simulink model "hwTarget"  (R2020b)
settings: Solver=VariableStepAuto  StartTime=0.0  StopTime=Ts  RelTol=1e-3
InitFcn:
  | evalin('base','pixelcontrolbus');
  | 
  | ROWS = 480;
  | COLS = 752;
  | 
  | OFFSET = 3;
  | imagesToRead = 20;
  | Ts = (imagesToRead + OFFSET) * 2;
  | 
  | inputNums = [1:imagesToRead];
  | 
  | MagThrL = 7;
  | MagThrS = 3;
  | SegMaxLength = 630;
  | 
  | NUM_OF_BITS = 32;
  | MSB = NUM_OF_BITS-1;
  | cap_1 = fixdt(0,NUM_OF_BITS,NUM_OF_BITS-1);
  | cap_2 = fixdt(0,NUM_OF_BITS,NUM_OF_BITS-2);
  | 
  | CORDIC_LUT_DT_1 = fixdt(1, NUM_OF_BITS, NUM_OF_BITS-2);
  | CORDIC_LUT_DT_2 = fixdt(1, NUM_OF_BITS, NUM_OF_BITS-1);
  | CORDIC_LUT_DT_3 = fixdt(1, NUM_OF_BITS, NUM_OF_BITS);
  | CORDIC_LUT_DT_4 = fixdt(1, NUM_OF_BITS, NUM_OF_BITS+1);
  | CORDIC_LUT_DT_5 = fixdt(1, NUM_OF_BITS, NUM_OF_BITS+1);
  | CORDIC_LUT_DT_6 = fixdt(1, NUM_OF_BITS, NUM_OF_BITS+2);
  | CORDIC_LUT_DT_7 = fixdt(1, NUM_OF_BITS, NUM_OF_BITS+3);
  | CORDIC_LUT_DT_8 = fixdt(1, NUM_OF_BITS, NUM_OF_BITS+4);
  | CORDIC_LUT_DT_9 = fixdt(1, NUM_OF_BITS, NUM_OF_BITS+5);
  | CORDIC_LUT_DT_10 = fixdt(1, NUM_OF_BITS, NUM_OF_BITS+6);
  | CORDIC_LUT_DT_11 = fixdt(1, NUM_OF_BITS, NUM_OF_BITS+7);
  | CORDIC_LUT_DT_12 = fixdt(1, NUM_OF_BITS, NUM_OF_BITS+8);
  | 
  | RGB_DT = fixdt(0, 24, 0);
  | GRAY_DT = fixdt(0, 8, 0);
  | THETA_DT = fixdt(1, 16, 13);
  | MAG_DT = fixdt(0, 16, 15);
  | KIRCH_DT = fixdt(0, 12, 0);
undefined symbols (not defined in the file or in its folder): bufferInit, bufferSize
libraries: hdlsllib x86, simulink x6, visionhdlstatistics x4, visionhdlio x2, visionhdlutilities x1
(part 2 of 3)

== system hwTarget/hwTarget/Kirsch Operation North/Kirch Filter North/Kirch Filter ==
  data_in : Inport
  Enable : EnablePort
  Abs : Abs  OutDataTypeStr=fixdt(0,12,0)
  Delay{,1..3,5} (5 alike) : Delay  DelayLength=1
  Gain1 : Gain  Gain=3  OutDataTypeStr=fixdt(0,13,0)
  Multiply : Gain  Gain=5  OutDataTypeStr=fixdt(0,13,0)
  Subtract : Sum  Inputs=+-  OutDataTypeStr=fixdt(1,13,0)
  Sum : Sum  Inputs=+  OutDataTypeStr=fixdt(0,10,0)
  Sum1 : Sum  Inputs=+  OutDataTypeStr=fixdt(0,11,0)
  slicer : Subsystem
  Out1 : Outport
  wires:
  slicer/2(nThrees) -> Sum1/1
  slicer/1(Fives) -> Sum/1
  Sum/1 -> Delay1/1
  Delay/1 -> Gain1/1
  Delay1/1 -> Multiply/1
  Subtract/1 -> Abs/1
  Sum1/1 -> Delay/1
  Abs/1 -> Delay5/1
  Delay2/1 -> Subtract/2
  Gain1/1 -> Delay2/1
  Delay3/1 -> Subtract/1
  Multiply/1 -> Delay3/1
  data_in/1 -> slicer/1(data_in)
  Delay5/1 -> Out1/1

== system hwTarget/hwTarget/Kirsch Operation North/Statistical Analysis/Latch ==
  note: Latch (Active low rst)
      | Ethan Tola
      | 04/03/2021
  D : Inport
  en : Inport  Port=2  OutMin=[0]  OutMax=[1]
  rstn : Inport  Port=3
  Constant : Constant  Value=0  OutDataTypeStr=Inherit: Inherit via back propagation  SampleTime=-1
  Data Type Duplicate : DataTypeDuplicate
  Memory : Memory  InheritSampleTime=on
  Switch : Switch  Criteria=u2 > Threshold
  Switch1 : Switch  Criteria=u2 > Threshold
  Q : Outport
  wires:
  Memory/1 -> Switch/3
  Switch/1 -> Data Type Duplicate/1, Switch1/1, Memory/1
  en/1 -> Switch/2
  D/1 -> Switch/1
  Switch1/1 -> Q/1
  rstn/1 -> Switch1/2
  Constant/1 -> Switch1/3, Data Type Duplicate/2

== system hwTarget/hwTarget/Kirsch Operation North/Statistical Analysis/Latch1 ==
  note: Latch (Active low rst)
      | Ethan Tola
      | 04/03/2021
  D : Inport
  en : Inport  Port=2  OutMin=[0]  OutMax=[1]
  rstn : Inport  Port=3
  Constant : Constant  Value=0  OutDataTypeStr=Inherit: Inherit via back propagation  SampleTime=-1
  Data Type Duplicate : DataTypeDuplicate
  Memory : Memory  InheritSampleTime=on
  Switch : Switch  Criteria=u2 > Threshold
  Switch1 : Switch  Criteria=u2 > Threshold
  Q : Outport
  wires:
  Memory/1 -> Switch/3
  Switch/1 -> Data Type Duplicate/1, Switch1/1, Memory/1
  en/1 -> Switch/2
  D/1 -> Switch/1
  Switch1/1 -> Q/1
  rstn/1 -> Switch1/2
  Constant/1 -> Switch1/3, Data Type Duplicate/2

== system hwTarget/hwTarget/Kirsch Operation Northwest/Binarize/Subsystem ==
  pixel : Inport
  mean : Inport  Port=2
  stddev : Inport  Port=3
  magThrL : Inport  Port=4
  magThrS : Inport  Port=5
  Enable : EnablePort
  Comparator : RelationalOperator  Operator=>  OutDataTypeStr=boolean  RndMeth=Simplest
  Comparator1 : RelationalOperator  Operator=>  OutDataTypeStr=boolean  RndMeth=Simplest
  Delay : Delay  DelayLength=1
  Delay1 : Delay  DelayLength=1
  Delay2 : Delay  DelayLength=1
  MagThrL : Subsystem
  MagThrS : Subsystem
  Out1 : Outport
  Out2 : Outport  Port=2
  wires:
  pixel/1 -> Delay2/1
  MagThrL/1(thresh) -> Delay1/1
  magThrS/1 -> MagThrS/3(dev_step)
  MagThrS/1(thresh) -> Delay/1
  magThrL/1 -> MagThrL/3(dev_step)
  mean/1 -> MagThrS/1(mean), MagThrL/1(mean)
  stddev/1 -> MagThrS/2(stddev), MagThrL/2(stddev)
  Comparator1/1 -> Out2/1
  Comparator/1 -> Out1/1
  Delay/1 -> Comparator1/2
  Delay1/1 -> Comparator/2
  Delay2/1 -> Comparator1/1, Comparator/1

== system hwTarget/hwTarget/Kirsch Operation Northwest/Kirch Filter North-West/Kirch Filter ==
  data_in : Inport
  Enable : EnablePort
  Abs : Abs  OutDataTypeStr=fixdt(0,12,0)
  Delay{,1..3,5} (5 alike) : Delay  DelayLength=1
  Gain1 : Gain  Gain=3  OutDataTypeStr=fixdt(0,13,0)
  Multiply : Gain  Gain=5  OutDataTypeStr=fixdt(0,13,0)
  Subtract : Sum  Inputs=+-  OutDataTypeStr=fixdt(1,13,0)
  Sum : Sum  Inputs=+  OutDataTypeStr=fixdt(0,10,0)
  Sum1 : Sum  Inputs=+  OutDataTypeStr=fixdt(0,11,0)
  slicer : Subsystem
  Out1 : Outport
  wires:
  Sum/1 -> Delay1/1
  Subtract/1 -> Abs/1
  Gain1/1 -> Delay2/1
  Multiply/1 -> Delay3/1
  slicer/2(nThrees) -> Sum1/1
  Sum1/1 -> Delay/1
  Delay3/1 -> Subtract/1
  Delay/1 -> Gain1/1
  Delay1/1 -> Multiply/1
  Abs/1 -> Delay5/1
  slicer/1(Fives) -> Sum/1
  Delay2/1 -> Subtract/2
  data_in/1 -> slicer/1(data_in)
  Delay5/1 -> Out1/1

== system hwTarget/hwTarget/Kirsch Operation Northwest/Statistical Analysis/Latch ==
  note: Latch (Active low rst)
      | Ethan Tola
      | 04/03/2021
  D : Inport
  en : Inport  Port=2  OutMin=[0]  OutMax=[1]
  rstn : Inport  Port=3
  Constant : Constant  Value=0  OutDataTypeStr=Inherit: Inherit via back propagation  SampleTime=-1
  Data Type Duplicate : DataTypeDuplicate
  Memory : Memory  InheritSampleTime=on
  Switch : Switch  Criteria=u2 > Threshold
  Switch1 : Switch  Criteria=u2 > Threshold
  Q : Outport
  wires:
  Memory/1 -> Switch/3
  Switch/1 -> Data Type Duplicate/1, Switch1/1, Memory/1
  en/1 -> Switch/2
  D/1 -> Switch/1
  Switch1/1 -> Q/1
  rstn/1 -> Switch1/2
  Constant/1 -> Switch1/3, Data Type Duplicate/2

== system hwTarget/hwTarget/Kirsch Operation Northwest/Statistical Analysis/Latch1 ==
  note: Latch (Active low rst)
      | Ethan Tola
      | 04/03/2021
  D : Inport
  en : Inport  Port=2  OutMin=[0]  OutMax=[1]
  rstn : Inport  Port=3
  Constant : Constant  Value=0  OutDataTypeStr=Inherit: Inherit via back propagation  SampleTime=-1
  Data Type Duplicate : DataTypeDuplicate
  Memory : Memory  InheritSampleTime=on
  Switch : Switch  Criteria=u2 > Threshold
  Switch1 : Switch  Criteria=u2 > Threshold
  Q : Outport
  wires:
  Memory/1 -> Switch/3
  Switch/1 -> Data Type Duplicate/1, Switch1/1, Memory/1
  en/1 -> Switch/2
  D/1 -> Switch/1
  Switch1/1 -> Q/1
  rstn/1 -> Switch1/2
  Constant/1 -> Switch1/3, Data Type Duplicate/2

== system hwTarget/hwTarget/Kirsch Operation Southwest/Binarize/Subsystem ==
  pixel : Inport
  mean : Inport  Port=2
  stddev : Inport  Port=3
  magThrL : Inport  Port=4
  magThrS : Inport  Port=5
  Enable : EnablePort
  Comparator : RelationalOperator  Operator=>  OutDataTypeStr=boolean  RndMeth=Simplest
  Comparator1 : RelationalOperator  Operator=>  OutDataTypeStr=boolean  RndMeth=Simplest
  Delay : Delay  DelayLength=1
  Delay1 : Delay  DelayLength=1
  Delay2 : Delay  DelayLength=1
  MagThrL : Subsystem
  MagThrS : Subsystem
  Out1 : Outport
  Out2 : Outport  Port=2
  wires:
  pixel/1 -> Delay2/1
  MagThrL/1(thresh) -> Delay1/1
  magThrS/1 -> MagThrS/3(dev_step)
  MagThrS/1(thresh) -> Delay/1
  magThrL/1 -> MagThrL/3(dev_step)
  mean/1 -> MagThrS/1(mean), MagThrL/1(mean)
  stddev/1 -> MagThrS/2(stddev), MagThrL/2(stddev)
  Comparator1/1 -> Out2/1
  Comparator/1 -> Out1/1
  Delay/1 -> Comparator1/2
  Delay1/1 -> Comparator/2
  Delay2/1 -> Comparator1/1, Comparator/1

== system hwTarget/hwTarget/Kirsch Operation Southwest/Kirch Filter South-West/Subsystem ==
  data_in : Inport
  Enable : EnablePort
  Abs : Abs  OutDataTypeStr=fixdt(0,12,0)
  Delay{,1..3,5} (5 alike) : Delay  DelayLength=1
  Gain1 : Gain  Gain=3  OutDataTypeStr=fixdt(0,13,0)
  Multiply : Gain  Gain=5  OutDataTypeStr=fixdt(0,13,0)
  Subtract : Sum  Inputs=+-  OutDataTypeStr=fixdt(1,13,0)
  Sum : Sum  Inputs=+  OutDataTypeStr=fixdt(0,10,0)
  Sum1 : Sum  Inputs=+  OutDataTypeStr=fixdt(0,11,0)
  slicer : Subsystem
  Out1 : Outport
  wires:
  Delay1/1 -> Multiply/1
  slicer/2(nThrees) -> Sum1/1
  Delay/1 -> Gain1/1
  Gain1/1 -> Delay2/1
  Delay3/1 -> Subtract/1
  Subtract/1 -> Abs/1
  slicer/1(Fives) -> Sum/1
  Multiply/1 -> Delay3/1
  Abs/1 -> Delay5/1
  Delay5/1 -> Out1/1
  Delay2/1 -> Subtract/2
  Sum/1 -> Delay1/1
  Sum1/1 -> Delay/1
  data_in/1 -> slicer/1(data_in)

== system hwTarget/hwTarget/Kirsch Operation Southwest/Statistical Analysis/Latch ==
  note: Latch (Active low rst)
      | Ethan Tola
      | 04/03/2021
  D : Inport
  en : Inport  Port=2  OutMin=[0]  OutMax=[1]
  rstn : Inport  Port=3
  Constant : Constant  Value=0  OutDataTypeStr=Inherit: Inherit via back propagation  SampleTime=-1
  Data Type Duplicate : DataTypeDuplicate
  Memory : Memory  InheritSampleTime=on
  Switch : Switch  Criteria=u2 > Threshold
  Switch1 : Switch  Criteria=u2 > Threshold
  Q : Outport
  wires:
  Memory/1 -> Switch/3
  Switch/1 -> Data Type Duplicate/1, Switch1/1, Memory/1
  en/1 -> Switch/2
  D/1 -> Switch/1
  Switch1/1 -> Q/1
  rstn/1 -> Switch1/2
  Constant/1 -> Switch1/3, Data Type Duplicate/2

== system hwTarget/hwTarget/Kirsch Operation Southwest/Statistical Analysis/Latch1 ==
  note: Latch (Active low rst)
      | Ethan Tola
      | 04/03/2021
  D : Inport
  en : Inport  Port=2  OutMin=[0]  OutMax=[1]
  rstn : Inport  Port=3
  Constant : Constant  Value=0  OutDataTypeStr=Inherit: Inherit via back propagation  SampleTime=-1
  Data Type Duplicate : DataTypeDuplicate
  Memory : Memory  InheritSampleTime=on
  Switch : Switch  Criteria=u2 > Threshold
  Switch1 : Switch  Criteria=u2 > Threshold
  Q : Outport
  wires:
  Memory/1 -> Switch/3
  Switch/1 -> Data Type Duplicate/1, Switch1/1, Memory/1
  en/1 -> Switch/2
  D/1 -> Switch/1
  Switch1/1 -> Q/1
  rstn/1 -> Switch1/2
  Constant/1 -> Switch1/3, Data Type Duplicate/2

== system hwTarget/hwTarget/Kirsch Operation West/Binarize/Subsystem ==
  pixel : Inport
  mean : Inport  Port=2
  stddev : Inport  Port=3
  magThrL : Inport  Port=4
  magThrS : Inport  Port=5
  Enable : EnablePort
  Comparator : RelationalOperator  Operator=>  OutDataTypeStr=boolean  RndMeth=Simplest
  Comparator1 : RelationalOperator  Operator=>  OutDataTypeStr=boolean  RndMeth=Simplest
  Delay : Delay  DelayLength=1
  Delay1 : Delay  DelayLength=1
  Delay2 : Delay  DelayLength=1
  MagThrL : Subsystem
  MagThrS : Subsystem
  Out1 : Outport
  Out2 : Outport  Port=2
  wires:
  pixel/1 -> Delay2/1
  MagThrL/1(thresh) -> Delay1/1
  magThrS/1 -> MagThrS/3(dev_step)
  MagThrS/1(thresh) -> Delay/1
  magThrL/1 -> MagThrL/3(dev_step)
  mean/1 -> MagThrS/1(mean), MagThrL/1(mean)
  stddev/1 -> MagThrS/2(stddev), MagThrL/2(stddev)
  Comparator1/1 -> Out2/1
  Comparator/1 -> Out1/1
  Delay/1 -> Comparator1/2
  Delay1/1 -> Comparator/2
  Delay2/1 -> Comparator1/1, Comparator/1

== system hwTarget/hwTarget/Kirsch Operation West/Kirch Filter West/Subsystem ==
  data_in : Inport
  Enable : EnablePort
  Abs : Abs  OutDataTypeStr=fixdt(0,12,0)
  Delay{,1..3,5} (5 alike) : Delay  DelayLength=1
  Gain1 : Gain  Gain=3  OutDataTypeStr=fixdt(0,13,0)
  Multiply : Gain  Gain=5  OutDataTypeStr=fixdt(0,13,0)
  Subtract : Sum  Inputs=+-  OutDataTypeStr=fixdt(1,13,0)
  Sum : Sum  Inputs=+  OutDataTypeStr=fixdt(0,10,0)
  Sum1 : Sum  Inputs=+  OutDataTypeStr=fixdt(0,11,0)
  slicer : Subsystem
  Out1 : Outport
  wires:
  Subtract/1 -> Abs/1
  Abs/1 -> Delay5/1
  Delay2/1 -> Subtract/2
  Multiply/1 -> Delay3/1
  Delay3/1 -> Subtract/1
  Delay1/1 -> Multiply/1
  slicer/1(Fives) -> Sum/1
  Delay/1 -> Gain1/1
  Sum1/1 -> Delay/1
  slicer/2(nThrees) -> Sum1/1
  Sum/1 -> Delay1/1
  Delay5/1 -> Out1/1
  Gain1/1 -> Delay2/1
  data_in/1 -> slicer/1(data_in)

== system hwTarget/hwTarget/Kirsch Operation West/Statistical Analysis/Latch ==
  note: Latch (Active low rst)
      | Ethan Tola
      | 04/03/2021
  D : Inport
  en : Inport  Port=2  OutMin=[0]  OutMax=[1]
  rstn : Inport  Port=3
  Constant : Constant  Value=0  OutDataTypeStr=Inherit: Inherit via back propagation  SampleTime=-1
  Data Type Duplicate : DataTypeDuplicate
  Memory : Memory  InheritSampleTime=on
  Switch : Switch  Criteria=u2 > Threshold
  Switch1 : Switch  Criteria=u2 > Threshold
  Q : Outport
  wires:
  Memory/1 -> Switch/3
  Switch/1 -> Data Type Duplicate/1, Switch1/1, Memory/1
  en/1 -> Switch/2
  D/1 -> Switch/1
  Switch1/1 -> Q/1
  rstn/1 -> Switch1/2
  Constant/1 -> Switch1/3, Data Type Duplicate/2

== system hwTarget/hwTarget/Kirsch Operation West/Statistical Analysis/Latch1 ==
  note: Latch (Active low rst)
      | Ethan Tola
      | 04/03/2021
  D : Inport
  en : Inport  Port=2  OutMin=[0]  OutMax=[1]
  rstn : Inport  Port=3
  Constant : Constant  Value=0  OutDataTypeStr=Inherit: Inherit via back propagation  SampleTime=-1
  Data Type Duplicate : DataTypeDuplicate
  Memory : Memory  InheritSampleTime=on
  Switch : Switch  Criteria=u2 > Threshold
  Switch1 : Switch  Criteria=u2 > Threshold
  Q : Outport
  wires:
  Memory/1 -> Switch/3
  Switch/1 -> Data Type Duplicate/1, Switch1/1, Memory/1
  en/1 -> Switch/2
  D/1 -> Switch/1
  Switch1/1 -> Q/1
  rstn/1 -> Switch1/2
  Constant/1 -> Switch1/3, Data Type Duplicate/2

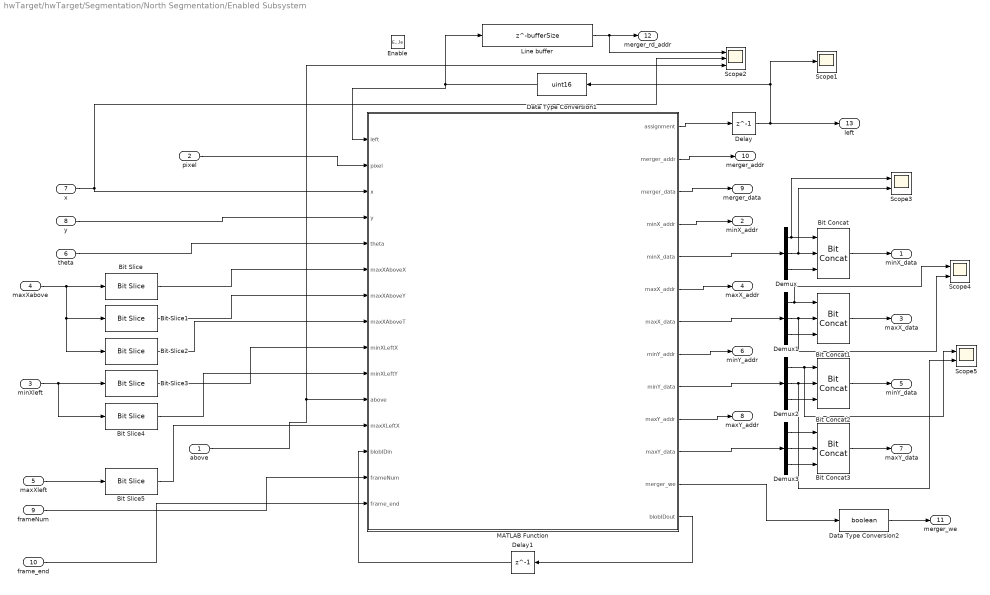
== system hwTarget/hwTarget/Segmentation/North Segmentation/Enabled Subsystem ==
  above : Inport
  pixel : Inport  Port=2
  minXleft : Inport  Port=3
  maxXabove : Inport  Port=4
  maxXleft : Inport  Port=5
  theta : Inport  Port=6
  x : Inport  Port=7
  y : Inport  Port=8
  frameNum : Inport  Port=9
  frame_end : Inport  Port=10
  Enable : EnablePort
  Bit Concat{,1..3} (4 alike) : hdlsllib/Logic and Bit Operations/Bit Concat  numInputs=3
  Bit Slice : hdlsllib/Logic and Bit Operations/Bit Slice  lidx=47  ridx=32
      settings: SourceProductBaseCode=SL
  Bit Slice1 : hdlsllib/Logic and Bit Operations/Bit Slice  lidx=31  ridx=16
      settings: SourceProductBaseCode=SL
  Bit Slice2 : hdlsllib/Logic and Bit Operations/Bit Slice  lidx=15  ridx=0
      settings: SourceProductBaseCode=SL
  Bit Slice3 : hdlsllib/Logic and Bit Operations/Bit Slice  lidx=47  ridx=32
      settings: SourceProductBaseCode=SL
  Bit Slice4 : hdlsllib/Logic and Bit Operations/Bit Slice  lidx=31  ridx=16
      settings: SourceProductBaseCode=SL
  Bit Slice5 : hdlsllib/Logic and Bit Operations/Bit Slice  lidx=47  ridx=32
      settings: SourceProductBaseCode=SL
  Data Type Conversion1 : DataTypeConversion  OutDataTypeStr=uint16
  Data Type Conversion2 : DataTypeConversion  OutDataTypeStr=boolean
  Delay : Delay  DelayLength=1  InitialCondition=0
  Delay1 : Delay  DelayLength=1  InitialCondition=1
  Demux{,1..3} (4 alike) : Demux  Outputs=3
  Line buffer : Delay  DelayLength=bufferSize  InitialCondition=bufferInit
  MATLAB Function : MATLAB Function  TreatAsAtomicUnit=on
  Scope1 : Scope
  Scope2 : Scope  NumInputPorts=3
  Scope3 : Scope  NumInputPorts=2
  Scope4 : Scope  NumInputPorts=2
  Scope5 : Scope  NumInputPorts=2
  minX_data : Outport  InitialOutput=0
  minX_addr : Outport  Port=2  InitialOutput=0
  maxX_data : Outport  Port=3  InitialOutput=0
  maxX_addr : Outport  Port=4  InitialOutput=0
  minY_data : Outport  Port=5  InitialOutput=0
  minY_addr : Outport  Port=6  InitialOutput=0
  maxY_data : Outport  Port=7  InitialOutput=0
  maxY_addr : Outport  Port=8  InitialOutput=0
  merger_data : Outport  Port=9  InitialOutput=0
  merger_addr : Outport  Port=10  InitialOutput=0
  merger_we : Outport  Port=11  InitialOutput=0
  merger_rd_addr : Outport  Port=12  InitialOutput=0
  left : Outport  Port=13  InitialOutput=0
  wires:
  Line buffer/1 -> Scope2/1, merger_rd_addr/1
  MATLAB Function/6(maxX_addr) -> maxX_addr/1
  MATLAB Function/4(minX_addr) -> minX_addr/1
  MATLAB Function/8(minY_addr) -> minY_addr/1
  MATLAB Function/10(maxY_addr) -> maxY_addr/1
  MATLAB Function/2(merger_addr) -> merger_addr/1
  Delay/1 -> Scope1/1, Data Type Conversion1/1, left/1
  MATLAB Function/1(assignment) -> Delay/1
  MATLAB Function/12(merger_we) -> Data Type Conversion2/1
  maxXabove/1 -> Bit Slice2/1, Bit Slice1/1, Bit Slice/1
  MATLAB Function/5(minX_data) -> Demux/1
  Bit Concat/1 -> minX_data/1
  Demux/1 -> Scope3/1, Bit Concat/1
  Demux/2 -> Scope3/2, Bit Concat/2
  Demux/3 -> Bit Concat/3
  MATLAB Function/7(maxX_data) -> Demux1/1
  Demux1/3 -> Bit Concat1/3
  Demux1/1 -> Scope4/1, Bit Concat1/1
  Demux1/2 -> Scope4/2, Bit Concat1/2
  Bit Concat1/1 -> maxX_data/1
  MATLAB Function/9(minY_data) -> Demux2/1
  Demux2/3 -> Bit Concat2/3
  Demux2/1 -> Scope5/1, Bit Concat2/1
  Demux2/2 -> Scope5/2, Bit Concat2/2
  Bit Concat2/1 -> minY_data/1
  MATLAB Function/11(maxY_data) -> Demux3/1
  Demux3/3 -> Bit Concat3/3
  Demux3/1 -> Bit Concat3/1
  Demux3/2 -> Bit Concat3/2
  Bit Concat3/1 -> maxY_data/1
  Data Type Conversion1/1 -> MATLAB Function/1(left), Line buffer/1
  pixel/1 -> MATLAB Function/2(pixel)
  x/1 -> Scope2/2, MATLAB Function/3(x)
  y/1 -> MATLAB Function/4(y)
  theta/1 -> MATLAB Function/5(theta)
  Bit Slice/1 -> MATLAB Function/6(maxXAboveX)
  Bit Slice1/1 -> MATLAB Function/7(maxXAboveY)
  Bit Slice2/1 -> MATLAB Function/8(maxXAboveT)
  Bit Slice3/1 -> MATLAB Function/9(minXLeftX)
  Bit Slice4/1 -> MATLAB Function/10(minXLeftY)
  Bit Slice5/1 -> MATLAB Function/12(maxXLeftX)
  above/1 -> Scope2/3, MATLAB Function/11(above)
  Data Type Conversion2/1 -> merger_we/1
  MATLAB Function/3(merger_data) -> merger_data/1
  Delay1/1 -> MATLAB Function/13(blobIDin)
  MATLAB Function/13(blobIDout) -> Delay1/1
  frameNum/1 -> MATLAB Function/14(frameNum)
  maxXleft/1 -> Bit Slice5/1
  minXleft/1 -> Bit Slice4/1, Bit Slice3/1
  frame_end/1 -> MATLAB Function/15(frame_end)

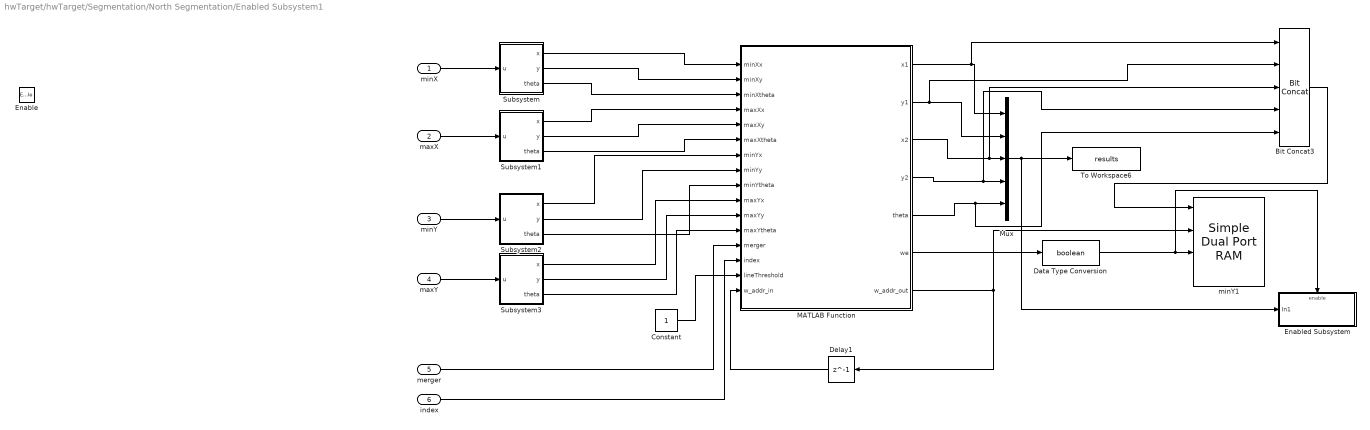
== system hwTarget/hwTarget/Segmentation/North Segmentation/Enabled Subsystem1 ==
  minX : Inport
  maxX : Inport  Port=2
  minY : Inport  Port=3
  maxY : Inport  Port=4
  merger : Inport  Port=5
  index : Inport  Port=6
  Enable : EnablePort
  Bit Concat3 : hdlsllib/Logic and Bit Operations/Bit Concat  numInputs=5
  Constant : Constant  OutDataTypeStr=uint16  SampleTime=-1
  Data Type Conversion : DataTypeConversion  OutDataTypeStr=boolean
  Delay1 : Delay  DelayLength=1  InitialCondition=0
  Enabled Subsystem : Subsystem  TreatAsAtomicUnit=on
  MATLAB Function : MATLAB Function  TreatAsAtomicUnit=on
  Mux : Mux  Inputs=5
  Subsystem : Subsystem
  Subsystem1 : Subsystem
  Subsystem2 : Subsystem
  Subsystem3 : Subsystem
  To Workspace6 : ToWorkspace  VariableName=results  SaveFormat=Timeseries  SampleTime=-1
  minY1 : hdlsllib/HDL RAMs/Simple Dual Port RAM  ram_size=16
      settings: SourceProductBaseCode=SL
  wires:
  minX/1 -> Subsystem/1(u)
  Subsystem/1(x) -> MATLAB Function/1(minXx)
  Subsystem/2(y) -> MATLAB Function/2(minXy)
  maxX/1 -> Subsystem1/1(u)
  minY/1 -> Subsystem2/1(u)
  Subsystem/3(theta) -> MATLAB Function/3(minXtheta)
  Subsystem1/1(x) -> MATLAB Function/4(maxXx)
  Subsystem1/2(y) -> MATLAB Function/5(maxXy)
  Subsystem1/3(theta) -> MATLAB Function/6(maxXtheta)
  Subsystem2/1(x) -> MATLAB Function/7(minYx)
  Subsystem2/2(y) -> MATLAB Function/8(minYy)
  Subsystem2/3(theta) -> MATLAB Function/9(minYtheta)
  maxY/1 -> Subsystem3/1(u)
  Subsystem3/1(x) -> MATLAB Function/10(maxYx)
  Subsystem3/2(y) -> MATLAB Function/11(maxYy)
  Subsystem3/3(theta) -> MATLAB Function/12(maxYtheta)
  merger/1 -> MATLAB Function/13(merger)
  index/1 -> MATLAB Function/14(index)
  Constant/1 -> MATLAB Function/15(lineThreshold)
  MATLAB Function/1(x1) -> Bit Concat3/1, Mux/1
  MATLAB Function/2(y1) -> Bit Concat3/2, Mux/2
  MATLAB Function/3(x2) -> Bit Concat3/3, Mux/3
  MATLAB Function/4(y2) -> Bit Concat3/4, Mux/4
  MATLAB Function/5(theta) -> Bit Concat3/5, Mux/5
  Mux/1 -> Enabled Subsystem/1(In1), To Workspace6/1
  MATLAB Function/7(w_addr_out) -> minY1/2, Delay1/1
  Delay1/1 -> MATLAB Function/16(w_addr_in)
  MATLAB Function/6(we) -> Data Type Conversion/1
  Bit Concat3/1 -> minY1/1
  Data Type Conversion/1 -> Enabled Subsystem/Enable, minY1/3

== system hwTarget/hwTarget/Segmentation/North Segmentation/Subsystem1 ==
  enable : Inport
  Constant : Constant  OutDataTypeStr=fixdt(0,10,0)  SampleTime=-1
  Delay2 : Delay  DelayLength=1  InitialCondition=1  ShowEnablePort=on
      settings: InputPortMap=u0,e6
  Sum : Sum  Inputs=|++  OutDataTypeStr=uint16
  counter : Outport
  wires:
  enable/1 -> Delay2/2
  Delay2/1 -> Sum/1
  Constant/1 -> Sum/2
  Sum/1 -> Delay2/1, counter/1  "blobID"

== system hwTarget/hwTarget/Segmentation/North Segmentation/Subsystem2 ==
  reset : Inport
  Constant : Constant  OutDataTypeStr=fixdt(0,10,0)  SampleTime=-1
  Delay2 : Delay  DelayLength=1  InitialCondition=0  ExternalReset=Level
      settings: InputPortMap=u0,r5
  Sum : Sum  Inputs=|++  OutDataTypeStr=uint16
  counter : Outport
  wires:
  reset/1 -> Delay2/2
  Delay2/1 -> Sum/1
  Constant/1 -> Sum/2
  Sum/1 -> Delay2/1, counter/1  "blobID"

== system hwTarget/hwTarget/Segmentation/North Segmentation/Subsystem3 ==
  reset : Inport
  Constant : Constant  OutDataTypeStr=fixdt(0,10,0)  SampleTime=-1
  Delay2 : Delay  DelayLength=1  InitialCondition=0  ExternalReset=Level
      settings: InputPortMap=u0,r5
  Sum : Sum  Inputs=|++  OutDataTypeStr=uint16
  counter : Outport
  wires:
  Sum/1 -> counter/1, Delay2/1  "blobID"
  Constant/1 -> Sum/2
  Delay2/1 -> Sum/1
  reset/1 -> Delay2/2

== system hwTarget/hwTarget/Segmentation/North Segmentation/maxXWriteSwitch ==
  valid : Inport
  data_in : Inport  Port=2
  addr_in : Inport  Port=3
  we_in : Inport  Port=4
  Constant2 : Constant  OutDataTypeStr=boolean  SampleTime=-1
  Constant3 : Constant  Value=0  OutDataTypeStr=boolean  SampleTime=-1
  Counter Limited : simulink/Sources/Counter Limited  uplimit=1023  tsamp=-1
  Index Vector : MultiPortSwitch  DataPortOrder=Zero-based contiguous  Inputs=2  zeroidx=on
  Index Vector1 : MultiPortSwitch  DataPortOrder=Zero-based contiguous  Inputs=2  zeroidx=on
  Index Vector2 : MultiPortSwitch  DataPortOrder=Zero-based contiguous  Inputs=2  zeroidx=on
  data_out : Outport
  addr_out : Outport  Port=2
  we : Outport  Port=3
  wires:
  Constant2/1 -> Index Vector2/2
  Counter Limited/1 -> Index Vector1/2
  Constant3/1 -> Index Vector/2
  valid/1 -> Index Vector/1, Index Vector1/1, Index Vector2/1
  we_in/1 -> Index Vector2/3
  Index Vector2/1 -> we/1
  data_in/1 -> Index Vector/3
  addr_in/1 -> Index Vector1/3
  Index Vector1/1 -> addr_out/1
  Index Vector/1 -> data_out/1

== system hwTarget/hwTarget/Segmentation/North Segmentation/maxYWriteSwitch ==
  valid : Inport
  data_in : Inport  Port=2
  addr_in : Inport  Port=3
  we_in : Inport  Port=4
  Constant2 : Constant  OutDataTypeStr=boolean  SampleTime=-1
  Constant3 : Constant  Value=0  OutDataTypeStr=boolean  SampleTime=-1
  Counter Limited : simulink/Sources/Counter Limited  uplimit=1023  tsamp=-1
  Index Vector : MultiPortSwitch  DataPortOrder=Zero-based contiguous  Inputs=2  zeroidx=on
  Index Vector1 : MultiPortSwitch  DataPortOrder=Zero-based contiguous  Inputs=2  zeroidx=on
  Index Vector2 : MultiPortSwitch  DataPortOrder=Zero-based contiguous  Inputs=2  zeroidx=on
  data_out : Outport
  addr_out : Outport  Port=2
  we : Outport  Port=3
  wires:
  Constant2/1 -> Index Vector2/2
  Counter Limited/1 -> Index Vector1/2
  Constant3/1 -> Index Vector/2
  valid/1 -> Index Vector/1, Index Vector1/1, Index Vector2/1
  we_in/1 -> Index Vector2/3
  Index Vector2/1 -> we/1
  data_in/1 -> Index Vector/3
  addr_in/1 -> Index Vector1/3
  Index Vector1/1 -> addr_out/1
  Index Vector/1 -> data_out/1

== system hwTarget/hwTarget/Segmentation/North Segmentation/minXReadSwitch ==
  valid : Inport
  addr_in1 : Inport  Port=2
  frame_end : Inport  Port=3
  Index Vector : MultiPortSwitch  DataPortOrder=Zero-based contiguous  Inputs=2  zeroidx=on
  Subsystem1 : Subsystem
  addr_out : Outport
  wires:
  valid/1 -> Index Vector/1
  Index Vector/1 -> addr_out/1
  addr_in1/1 -> Index Vector/3
  frame_end/1 -> Subsystem1/1(reset)
  Subsystem1/1(counter) -> Index Vector/2

== system hwTarget/hwTarget/Segmentation/North Segmentation/minXReadSwitch1 ==
  valid : Inport
  addr_in1 : Inport  Port=2
  frame_end : Inport  Port=3
  Index Vector : MultiPortSwitch  DataPortOrder=Zero-based contiguous  Inputs=2  zeroidx=on
  Subsystem1 : Subsystem
  addr_out : Outport
  wires:
  valid/1 -> Index Vector/1
  Index Vector/1 -> addr_out/1
  addr_in1/1 -> Index Vector/3
  frame_end/1 -> Subsystem1/1(reset)
  Subsystem1/1(counter) -> Index Vector/2

== system hwTarget/hwTarget/Segmentation/North Segmentation/minXReadSwitch3 ==
  valid : Inport
  addr_in1 : Inport  Port=2
  frame_end : Inport  Port=3
  Index Vector : MultiPortSwitch  DataPortOrder=Zero-based contiguous  Inputs=2  zeroidx=on
  Subsystem1 : Subsystem
  addr_out : Outport
  wires:
  valid/1 -> Index Vector/1
  Index Vector/1 -> addr_out/1
  addr_in1/1 -> Index Vector/3
  frame_end/1 -> Subsystem1/1(reset)
  Subsystem1/1(counter) -> Index Vector/2

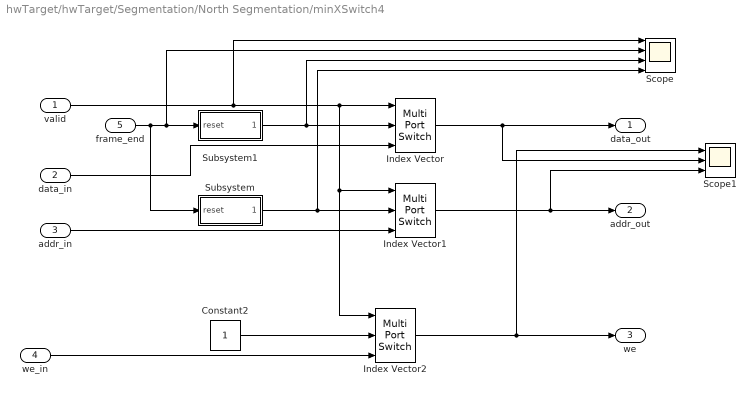
== system hwTarget/hwTarget/Segmentation/North Segmentation/minXSwitch4 ==
  valid : Inport
  data_in : Inport  Port=2
  addr_in : Inport  Port=3
  we_in : Inport  Port=4
  frame_end : Inport  Port=5
  Constant2 : Constant  OutDataTypeStr=boolean  SampleTime=-1
  Index Vector : MultiPortSwitch  DataPortOrder=Zero-based contiguous  Inputs=2  zeroidx=on
  Index Vector1 : MultiPortSwitch  DataPortOrder=Zero-based contiguous  Inputs=2  zeroidx=on
  Index Vector2 : MultiPortSwitch  DataPortOrder=Zero-based contiguous  Inputs=2  zeroidx=on
  Scope : Scope  NumInputPorts=4
  Scope1 : Scope  NumInputPorts=3
  Subsystem : Subsystem
  Subsystem1 : Subsystem
  data_out : Outport
  addr_out : Outport  Port=2
  we : Outport  Port=3
  wires:
  Index Vector/1 -> Scope1/2, data_out/1
  Index Vector1/1 -> Scope1/3, addr_out/1
  addr_in/1 -> Index Vector1/3
  data_in/1 -> Index Vector/3
  Index Vector2/1 -> Scope1/1, we/1
  we_in/1 -> Index Vector2/3
  valid/1 -> Scope/1, Index Vector2/1, Index Vector1/1, Index Vector/1
  Subsystem1/1(counter) -> Scope/3, Index Vector/2
  Subsystem/1(counter) -> Scope/4, Index Vector1/2
  Constant2/1 -> Index Vector2/2
  frame_end/1 -> Subsystem/1(reset), Scope/2, Subsystem1/1(reset)

== system hwTarget/hwTarget/Segmentation/North Segmentation/minXWriteSwitch ==
  valid : Inport
  data_in : Inport  Port=2
  addr_in : Inport  Port=3
  we_in : Inport  Port=4
  Constant2 : Constant  OutDataTypeStr=boolean  SampleTime=-1
  Constant3 : Constant  Value=0  OutDataTypeStr=boolean  SampleTime=-1
  Counter Limited : simulink/Sources/Counter Limited  uplimit=1023  tsamp=-1
  Index Vector : MultiPortSwitch  DataPortOrder=Zero-based contiguous  Inputs=2  zeroidx=on
  Index Vector1 : MultiPortSwitch  DataPortOrder=Zero-based contiguous  Inputs=2  zeroidx=on
  Index Vector2 : MultiPortSwitch  DataPortOrder=Zero-based contiguous  Inputs=2  zeroidx=on
  data_out : Outport
  addr_out : Outport  Port=2
  we : Outport  Port=3
  wires:
  Constant2/1 -> Index Vector2/2
  Counter Limited/1 -> Index Vector1/2
  Constant3/1 -> Index Vector/2
  valid/1 -> Index Vector/1, Index Vector1/1, Index Vector2/1
  we_in/1 -> Index Vector2/3
  Index Vector2/1 -> we/1
  data_in/1 -> Index Vector/3
  addr_in/1 -> Index Vector1/3
  Index Vector1/1 -> addr_out/1
  Index Vector/1 -> data_out/1

== system hwTarget/hwTarget/Segmentation/North Segmentation/minYWriteSwitch ==
  valid : Inport
  data_in : Inport  Port=2
  addr_in : Inport  Port=3
  we_in : Inport  Port=4
  Constant2 : Constant  OutDataTypeStr=boolean  SampleTime=-1
  Constant3 : Constant  Value=0  OutDataTypeStr=boolean  SampleTime=-1
  Counter Limited : simulink/Sources/Counter Limited  uplimit=1023  tsamp=-1
  Index Vector : MultiPortSwitch  DataPortOrder=Zero-based contiguous  Inputs=2  zeroidx=on
  Index Vector1 : MultiPortSwitch  DataPortOrder=Zero-based contiguous  Inputs=2  zeroidx=on
  Index Vector2 : MultiPortSwitch  DataPortOrder=Zero-based contiguous  Inputs=2  zeroidx=on
  data_out : Outport
  addr_out : Outport  Port=2
  we : Outport  Port=3
  wires:
  Index Vector/1 -> data_out/1
  Index Vector1/1 -> addr_out/1
  addr_in/1 -> Index Vector1/3
  data_in/1 -> Index Vector/3
  Index Vector2/1 -> we/1
  we_in/1 -> Index Vector2/3
  valid/1 -> Index Vector2/1, Index Vector1/1, Index Vector/1
  Constant3/1 -> Index Vector/2
  Counter Limited/1 -> Index Vector1/2
  Constant2/1 -> Index Vector2/2

== system hwTarget/hwTarget/CordicAtan/CORDIC Algorithm/Iteration_1/n_zsign ==
  signof : Inport
  base : Inport  Port=2
  Bit Slice : hdlsllib/Logic and Bit Operations/Bit Slice  lidx=MSB  ridx=MSB
      settings: SourceProductBaseCode=SL
  Switch : Switch  Criteria=u2 > Threshold
  Unary Minus : UnaryMinus
  out : Outport
  wires:
  Bit Slice/1 -> Switch/2
  signof/1 -> Bit Slice/1
  base/1 -> Switch/1, Unary Minus/1
  Switch/1 -> out/1
  Unary Minus/1 -> Switch/3

== system hwTarget/hwTarget/CordicAtan/CORDIC Algorithm/Iteration_1/n_zsign1 ==
  signof : Inport
  base : Inport  Port=2
  Bit Slice : hdlsllib/Logic and Bit Operations/Bit Slice  lidx=MSB  ridx=MSB
      settings: SourceProductBaseCode=SL
  Switch : Switch  Criteria=u2 > Threshold
  Unary Minus : UnaryMinus
  out : Outport
  wires:
  Bit Slice/1 -> Switch/2
  signof/1 -> Bit Slice/1
  base/1 -> Switch/1, Unary Minus/1
  Switch/1 -> out/1
  Unary Minus/1 -> Switch/3

== system hwTarget/hwTarget/CordicAtan/CORDIC Algorithm/Iteration_1/zsign ==
  signof : Inport
  base : Inport  Port=2
  Bit Slice : hdlsllib/Logic and Bit Operations/Bit Slice  lidx=MSB  ridx=MSB
      settings: SourceProductBaseCode=SL
  Switch : Switch  Criteria=u2 > Threshold
  Unary Minus : UnaryMinus
  out : Outport
  wires:
  signof/1 -> Bit Slice/1
  Bit Slice/1 -> Switch/2
  base/1 -> Switch/3, Unary Minus/1
  Switch/1 -> out/1
  Unary Minus/1 -> Switch/1

== system hwTarget/hwTarget/CordicAtan/CORDIC Algorithm/Iteration_10/X_Logic ==
  xo : Inport
  yo : Inport  Port=2
  Add2 : Sum
  Bit Shift : hdlsllib/Logic and Bit Operations/Bit Shift  mode=Shift Right Arithmetic  N=9
  zsign : Subsystem
  x : Outport
  wires:
  yo/1 -> zsign/1(signof), Bit Shift/1
  Bit Shift/1 -> zsign/2(base)
  xo/1 -> Add2/1
  Add2/1 -> x/1
  zsign/1(out) -> Add2/2  "xo"

== system hwTarget/hwTarget/CordicAtan/CORDIC Algorithm/Iteration_10/Y_Logic ==
  xo : Inport
  yo : Inport  Port=2
  Add1 : Sum
  Bit Shift : hdlsllib/Logic and Bit Operations/Bit Shift  mode=Shift Right Arithmetic  N=9
  n_zsign : Subsystem
  y : Outport
  wires:
  Bit Shift/1 -> n_zsign/2(base)
  n_zsign/1(out) -> Add1/2
  Add1/1 -> y/1
  xo/1 -> Bit Shift/1
  yo/1 -> n_zsign/1(signof), Add1/1

== system hwTarget/hwTarget/CordicAtan/CORDIC Algorithm/Iteration_10/n_zsign ==
  signof : Inport
  base : Inport  Port=2
  Bit Slice : hdlsllib/Logic and Bit Operations/Bit Slice  lidx=MSB  ridx=MSB
      settings: SourceProductBaseCode=SL
  Switch : Switch  Criteria=u2 > Threshold
  Unary Minus : UnaryMinus
  out : Outport
  wires:
  Bit Slice/1 -> Switch/2
  signof/1 -> Bit Slice/1
  base/1 -> Switch/1, Unary Minus/1
  Switch/1 -> out/1
  Unary Minus/1 -> Switch/3

== system hwTarget/hwTarget/CordicAtan/CORDIC Algorithm/Iteration_2/X_Logic ==
  xo : Inport
  yo : Inport  Port=2
  Add2 : Sum
  Bit Shift : hdlsllib/Logic and Bit Operations/Bit Shift  mode=Shift Right Arithmetic  N=1
  zsign1 : Subsystem
  x : Outport
  wires:
  yo/1 -> zsign1/1(signof), Bit Shift/1
  Bit Shift/1 -> zsign1/2(base)
  xo/1 -> Add2/1
  Add2/1 -> x/1
  zsign1/1(out) -> Add2/2  "xo"

== system hwTarget/hwTarget/CordicAtan/CORDIC Algorithm/Iteration_2/Y_Logic ==
  xo : Inport
  yo : Inport  Port=2
  Add1 : Sum
  Bit Shift : hdlsllib/Logic and Bit Operations/Bit Shift  mode=Shift Right Arithmetic  N=1
  n_zsign : Subsystem
  y : Outport
  wires:
  Bit Shift/1 -> n_zsign/2(base)
  n_zsign/1(out) -> Add1/2
  Add1/1 -> y/1
  xo/1 -> Bit Shift/1
  yo/1 -> n_zsign/1(signof), Add1/1

== system hwTarget/hwTarget/CordicAtan/CORDIC Algorithm/Iteration_2/n_zsign ==
  signof : Inport
  base : Inport  Port=2
  Bit Slice : hdlsllib/Logic and Bit Operations/Bit Slice  lidx=MSB  ridx=MSB
      settings: SourceProductBaseCode=SL
  Switch : Switch  Criteria=u2 > Threshold
  Unary Minus : UnaryMinus
  out : Outport
  wires:
  Bit Slice/1 -> Switch/2
  signof/1 -> Bit Slice/1
  base/1 -> Switch/1, Unary Minus/1
  Switch/1 -> out/1
  Unary Minus/1 -> Switch/3

== system hwTarget/hwTarget/CordicAtan/CORDIC Algorithm/Iteration_3/X_Logic ==
  xo : Inport
  yo : Inport  Port=2
  Add2 : Sum
  Bit Shift : hdlsllib/Logic and Bit Operations/Bit Shift  mode=Shift Right Arithmetic  N=2
  zsign : Subsystem
  x : Outport
  wires:
  yo/1 -> zsign/1(signof), Bit Shift/1
  Bit Shift/1 -> zsign/2(base)
  xo/1 -> Add2/1
  Add2/1 -> x/1
  zsign/1(out) -> Add2/2  "xo"

== system hwTarget/hwTarget/CordicAtan/CORDIC Algorithm/Iteration_3/Y_Logic ==
  xo : Inport
  yo : Inport  Port=2
  Add1 : Sum
  Bit Shift : hdlsllib/Logic and Bit Operations/Bit Shift  mode=Shift Right Arithmetic  N=2
  n_zsign : Subsystem
  y : Outport
  wires:
  Bit Shift/1 -> n_zsign/2(base)
  n_zsign/1(out) -> Add1/2
  Add1/1 -> y/1
  xo/1 -> Bit Shift/1
  yo/1 -> n_zsign/1(signof), Add1/1

== system hwTarget/hwTarget/CordicAtan/CORDIC Algorithm/Iteration_3/n_zsign ==
  signof : Inport
  base : Inport  Port=2
  Bit Slice : hdlsllib/Logic and Bit Operations/Bit Slice  lidx=MSB  ridx=MSB
      settings: SourceProductBaseCode=SL
  Switch : Switch  Criteria=u2 > Threshold
  Unary Minus : UnaryMinus
  out : Outport
  wires:
  Bit Slice/1 -> Switch/2
  signof/1 -> Bit Slice/1
  base/1 -> Switch/1, Unary Minus/1
  Switch/1 -> out/1
  Unary Minus/1 -> Switch/3

== system hwTarget/hwTarget/CordicAtan/CORDIC Algorithm/Iteration_4/X_Logic ==
  xo : Inport
  yo : Inport  Port=2
  Add2 : Sum
  Bit Shift : hdlsllib/Logic and Bit Operations/Bit Shift  mode=Shift Right Arithmetic  N=3
  zsign : Subsystem
  x : Outport
  wires:
  yo/1 -> zsign/1(signof), Bit Shift/1
  Bit Shift/1 -> zsign/2(base)
  xo/1 -> Add2/1
  Add2/1 -> x/1
  zsign/1(out) -> Add2/2  "xo"

== system hwTarget/hwTarget/CordicAtan/CORDIC Algorithm/Iteration_4/Y_Logic ==
  xo : Inport
  yo : Inport  Port=2
  Add1 : Sum
  Bit Shift : hdlsllib/Logic and Bit Operations/Bit Shift  mode=Shift Right Arithmetic  N=3
  n_zsign : Subsystem
  y : Outport
  wires:
  Bit Shift/1 -> n_zsign/2(base)
  n_zsign/1(out) -> Add1/2
  Add1/1 -> y/1
  xo/1 -> Bit Shift/1
  yo/1 -> n_zsign/1(signof), Add1/1

== system hwTarget/hwTarget/CordicAtan/CORDIC Algorithm/Iteration_4/n_zsign ==
  signof : Inport
  base : Inport  Port=2
  Bit Slice : hdlsllib/Logic and Bit Operations/Bit Slice  lidx=MSB  ridx=MSB
      settings: SourceProductBaseCode=SL
  Switch : Switch  Criteria=u2 > Threshold
  Unary Minus : UnaryMinus
  out : Outport
  wires:
  Bit Slice/1 -> Switch/2
  signof/1 -> Bit Slice/1
  base/1 -> Switch/1, Unary Minus/1
  Switch/1 -> out/1
  Unary Minus/1 -> Switch/3

== system hwTarget/hwTarget/CordicAtan/CORDIC Algorithm/Iteration_5/X_Logic ==
  xo : Inport
  yo : Inport  Port=2
  Add2 : Sum
  Bit Shift : hdlsllib/Logic and Bit Operations/Bit Shift  mode=Shift Right Arithmetic  N=4
  zsign : Subsystem
  x : Outport
  wires:
  yo/1 -> zsign/1(signof), Bit Shift/1
  Bit Shift/1 -> zsign/2(base)
  xo/1 -> Add2/1
  Add2/1 -> x/1
  zsign/1(out) -> Add2/2  "xo"

== system hwTarget/hwTarget/CordicAtan/CORDIC Algorithm/Iteration_5/Y_Logic ==
  xo : Inport
  yo : Inport  Port=2
  Add1 : Sum
  Bit Shift : hdlsllib/Logic and Bit Operations/Bit Shift  mode=Shift Right Arithmetic  N=4
  n_zsign : Subsystem
  y : Outport
  wires:
  Bit Shift/1 -> n_zsign/2(base)
  n_zsign/1(out) -> Add1/2
  Add1/1 -> y/1
  xo/1 -> Bit Shift/1
  yo/1 -> n_zsign/1(signof), Add1/1

== system hwTarget/hwTarget/CordicAtan/CORDIC Algorithm/Iteration_5/n_zsign ==
  signof : Inport
  base : Inport  Port=2
  Bit Slice : hdlsllib/Logic and Bit Operations/Bit Slice  lidx=MSB  ridx=MSB
      settings: SourceProductBaseCode=SL
  Switch : Switch  Criteria=u2 > Threshold
  Unary Minus : UnaryMinus
  out : Outport
  wires:
  Bit Slice/1 -> Switch/2
  signof/1 -> Bit Slice/1
  base/1 -> Switch/1, Unary Minus/1
  Switch/1 -> out/1
  Unary Minus/1 -> Switch/3

== system hwTarget/hwTarget/CordicAtan/CORDIC Algorithm/Iteration_6/X_Logic ==
  xo : Inport
  yo : Inport  Port=2
  Add2 : Sum
  Bit Shift : hdlsllib/Logic and Bit Operations/Bit Shift  mode=Shift Right Arithmetic  N=5
  zsign : Subsystem
  x : Outport
  wires:
  yo/1 -> zsign/1(signof), Bit Shift/1
  Bit Shift/1 -> zsign/2(base)
  xo/1 -> Add2/1
  Add2/1 -> x/1
  zsign/1(out) -> Add2/2  "xo"

== system hwTarget/hwTarget/CordicAtan/CORDIC Algorithm/Iteration_6/Y_Logic ==
  xo : Inport
  yo : Inport  Port=2
  Add1 : Sum
  Bit Shift : hdlsllib/Logic and Bit Operations/Bit Shift  mode=Shift Right Arithmetic  N=5
  n_zsign : Subsystem
  y : Outport
  wires:
  Bit Shift/1 -> n_zsign/2(base)
  n_zsign/1(out) -> Add1/2
  Add1/1 -> y/1
  xo/1 -> Bit Shift/1
  yo/1 -> n_zsign/1(signof), Add1/1

== system hwTarget/hwTarget/CordicAtan/CORDIC Algorithm/Iteration_6/n_zsign ==
  signof : Inport
  base : Inport  Port=2
  Bit Slice : hdlsllib/Logic and Bit Operations/Bit Slice  lidx=MSB  ridx=MSB
      settings: SourceProductBaseCode=SL
  Switch : Switch  Criteria=u2 > Threshold
  Unary Minus : UnaryMinus
  out : Outport
  wires:
  Bit Slice/1 -> Switch/2
  signof/1 -> Bit Slice/1
  base/1 -> Switch/1, Unary Minus/1
  Switch/1 -> out/1
  Unary Minus/1 -> Switch/3

== system hwTarget/hwTarget/CordicAtan/CORDIC Algorithm/Iteration_7/X_Logic ==
  xo : Inport
  yo : Inport  Port=2
  Add2 : Sum
  Bit Shift : hdlsllib/Logic and Bit Operations/Bit Shift  mode=Shift Right Arithmetic  N=6
  zsign : Subsystem
  x : Outport
  wires:
  yo/1 -> zsign/1(signof), Bit Shift/1
  Bit Shift/1 -> zsign/2(base)
  xo/1 -> Add2/1
  Add2/1 -> x/1
  zsign/1(out) -> Add2/2  "xo"

== system hwTarget/hwTarget/CordicAtan/CORDIC Algorithm/Iteration_7/Y_Logic ==
  xo : Inport
  yo : Inport  Port=2
  Add1 : Sum
  Bit Shift : hdlsllib/Logic and Bit Operations/Bit Shift  mode=Shift Right Arithmetic  N=6
  n_zsign : Subsystem
  y : Outport
  wires:
  Bit Shift/1 -> n_zsign/2(base)
  n_zsign/1(out) -> Add1/2
  Add1/1 -> y/1
  xo/1 -> Bit Shift/1
  yo/1 -> n_zsign/1(signof), Add1/1

== system hwTarget/hwTarget/CordicAtan/CORDIC Algorithm/Iteration_7/n_zsign ==
  signof : Inport
  base : Inport  Port=2
  Bit Slice : hdlsllib/Logic and Bit Operations/Bit Slice  lidx=MSB  ridx=MSB
      settings: SourceProductBaseCode=SL
  Switch : Switch  Criteria=u2 > Threshold
  Unary Minus : UnaryMinus
  out : Outport
  wires:
  Bit Slice/1 -> Switch/2
  signof/1 -> Bit Slice/1
  base/1 -> Switch/1, Unary Minus/1
  Switch/1 -> out/1
  Unary Minus/1 -> Switch/3

== system hwTarget/hwTarget/CordicAtan/CORDIC Algorithm/Iteration_8/X_Logic ==
  xo : Inport
  yo : Inport  Port=2
  Add2 : Sum
  Bit Shift : hdlsllib/Logic and Bit Operations/Bit Shift  mode=Shift Right Arithmetic  N=7
  zsign : Subsystem
  x : Outport
  wires:
  yo/1 -> zsign/1(signof), Bit Shift/1
  Bit Shift/1 -> zsign/2(base)
  xo/1 -> Add2/1
  Add2/1 -> x/1
  zsign/1(out) -> Add2/2  "xo"

== system hwTarget/hwTarget/CordicAtan/CORDIC Algorithm/Iteration_8/Y_Logic ==
  xo : Inport
  yo : Inport  Port=2
  Add1 : Sum
  Bit Shift : hdlsllib/Logic and Bit Operations/Bit Shift  mode=Shift Right Arithmetic  N=7
  n_zsign : Subsystem
  y : Outport
  wires:
  Bit Shift/1 -> n_zsign/2(base)
  n_zsign/1(out) -> Add1/2
  Add1/1 -> y/1
  xo/1 -> Bit Shift/1
  yo/1 -> n_zsign/1(signof), Add1/1

== system hwTarget/hwTarget/CordicAtan/CORDIC Algorithm/Iteration_8/n_zsign ==
  signof : Inport
  base : Inport  Port=2
  Bit Slice : hdlsllib/Logic and Bit Operations/Bit Slice  lidx=MSB  ridx=MSB
      settings: SourceProductBaseCode=SL
  Switch : Switch  Criteria=u2 > Threshold
  Unary Minus : UnaryMinus
  out : Outport
  wires:
  Bit Slice/1 -> Switch/2
  signof/1 -> Bit Slice/1
  base/1 -> Switch/1, Unary Minus/1
  Switch/1 -> out/1
  Unary Minus/1 -> Switch/3

== system hwTarget/hwTarget/CordicAtan/CORDIC Algorithm/Iteration_9/X_Logic ==
  xo : Inport
  yo : Inport  Port=2
  Add2 : Sum
  Bit Shift : hdlsllib/Logic and Bit Operations/Bit Shift  mode=Shift Right Arithmetic  N=8
  zsign : Subsystem
  x : Outport
  wires:
  yo/1 -> zsign/1(signof), Bit Shift/1
  Bit Shift/1 -> zsign/2(base)
  xo/1 -> Add2/1
  Add2/1 -> x/1
  zsign/1(out) -> Add2/2  "xo"

== system hwTarget/hwTarget/CordicAtan/CORDIC Algorithm/Iteration_9/Y_Logic ==
  xo : Inport
  yo : Inport  Port=2
  Add1 : Sum
  Bit Shift : hdlsllib/Logic and Bit Operations/Bit Shift  mode=Shift Right Arithmetic  N=8
  n_zsign : Subsystem
  y : Outport
  wires:
  Bit Shift/1 -> n_zsign/2(base)
  n_zsign/1(out) -> Add1/2
  Add1/1 -> y/1
  xo/1 -> Bit Shift/1
  yo/1 -> n_zsign/1(signof), Add1/1

== system hwTarget/hwTarget/CordicAtan/CORDIC Algorithm/Iteration_9/n_zsign ==
  signof : Inport
  base : Inport  Port=2
  Bit Slice : hdlsllib/Logic and Bit Operations/Bit Slice  lidx=MSB  ridx=MSB
      settings: SourceProductBaseCode=SL
  Switch : Switch  Criteria=u2 > Threshold
  Unary Minus : UnaryMinus
  out : Outport
  wires:
  Bit Slice/1 -> Switch/2
  signof/1 -> Bit Slice/1
  base/1 -> Switch/1, Unary Minus/1
  Switch/1 -> out/1
  Unary Minus/1 -> Switch/3

== system hwTarget/hwTarget/CordicAtan/CORDIC Algorithm/Setup_Stage/n_zsign ==
  signof : Inport
  base : Inport  Port=2
  Bit Slice : hdlsllib/Logic and Bit Operations/Bit Slice  lidx=MSB  ridx=MSB
      settings: SourceProductBaseCode=SL
  Switch : Switch  Criteria=u2 > Threshold
  Unary Minus : UnaryMinus
  out : Outport
  wires:
  Bit Slice/1 -> Switch/2
  signof/1 -> Bit Slice/1
  base/1 -> Switch/1, Unary Minus/1
  Switch/1 -> out/1
  Unary Minus/1 -> Switch/3

== system hwTarget/hwTarget/CordicAtan/CORDIC Algorithm/Setup_Stage/n_zsign1 ==
  signof : Inport
  base : Inport  Port=2
  Bit Slice : hdlsllib/Logic and Bit Operations/Bit Slice  lidx=MSB  ridx=MSB
      settings: SourceProductBaseCode=SL
  Switch : Switch  Criteria=u2 > Threshold
  Unary Minus : UnaryMinus
  out : Outport
  wires:
  Bit Slice/1 -> Switch/2
  signof/1 -> Bit Slice/1
  base/1 -> Switch/1, Unary Minus/1
  Switch/1 -> out/1
  Unary Minus/1 -> Switch/3

== system hwTarget/hwTarget/CordicAtan/CORDIC Algorithm/Setup_Stage/n_zsign2 ==
  signof : Inport
  base : Inport  Port=2
  Bit Slice : hdlsllib/Logic and Bit Operations/Bit Slice  lidx=MSB  ridx=MSB
      settings: SourceProductBaseCode=SL
  Switch : Switch  Criteria=u2 > Threshold
  Unary Minus : UnaryMinus
  out : Outport
  wires:
  Bit Slice/1 -> Switch/2
  signof/1 -> Bit Slice/1
  base/1 -> Switch/1, Unary Minus/1
  Switch/1 -> out/1
  Unary Minus/1 -> Switch/3

== system hwTarget/hwTarget/CordicAtan/CORDIC Algorithm/Setup_Stage/zsign ==
  signof : Inport
  base : Inport  Port=2
  Bit Slice : hdlsllib/Logic and Bit Operations/Bit Slice  lidx=MSB  ridx=MSB
      settings: SourceProductBaseCode=SL
  Switch : Switch  Criteria=u2 > Threshold
  Unary Minus : UnaryMinus
  out : Outport
  wires:
  signof/1 -> Bit Slice/1
  Bit Slice/1 -> Switch/2
  base/1 -> Switch/3, Unary Minus/1
  Switch/1 -> out/1
  Unary Minus/1 -> Switch/1

== system hwTarget/hwTarget/GaussianFilter/Symmetric Filter/Row Filter1/Symmetry ==
  data_in : Inport
  Add : Sum  Inputs=|++  AccumDataTypeStr=cap_2  OutDataTypeStr=cap_2  RndMeth=Nearest
  Data Type Duplicate : DataTypeDuplicate
  Data Type Conversion : DataTypeConversion
  Demux : Demux  Outputs=3
  Mux : Mux  Inputs=2
  data_out : Outport
  wires:
  Add/1 -> Data Type Duplicate/1, Mux/1
  data_in/1 -> Demux/1
  Demux/3 -> Add/2
  Demux/1 -> Add/1
  Mux/1 -> data_out/1
  Demux/2 -> Data Type Conversion/1
  Data Type Conversion/1 -> Data Type Duplicate/2, Mux/2

== system hwTarget/hwTarget/GaussianFilter/Symmetric Filter/Row Filter2/Symmetry ==
  data_in : Inport
  Add : Sum  Inputs=|++  AccumDataTypeStr=cap_2  OutDataTypeStr=cap_2  RndMeth=Nearest
  Data Type Duplicate : DataTypeDuplicate
  Data Type Conversion : DataTypeConversion
  Demux : Demux  Outputs=3
  Mux : Mux  Inputs=2
  data_out : Outport
  wires:
  Add/1 -> Data Type Duplicate/1, Mux/1
  data_in/1 -> Demux/1
  Demux/3 -> Add/2
  Demux/1 -> Add/1
  Mux/1 -> data_out/1
  Demux/2 -> Data Type Conversion/1
  Data Type Conversion/1 -> Data Type Duplicate/2, Mux/2

== system hwTarget/hwTarget/GaussianFilter/Symmetric Filter/Row Filter3/Symmetry ==
  data_in : Inport
  Add : Sum  Inputs=|++  AccumDataTypeStr=cap_2  OutDataTypeStr=cap_2  RndMeth=Nearest
  Data Type Duplicate : DataTypeDuplicate
  Data Type Conversion : DataTypeConversion
  Demux : Demux  Outputs=3
  Mux : Mux  Inputs=2
  data_out : Outport
  wires:
  Add/1 -> Data Type Duplicate/1, Mux/1
  data_in/1 -> Demux/1
  Demux/3 -> Add/2
  Demux/1 -> Add/1
  Mux/1 -> data_out/1
  Demux/2 -> Data Type Conversion/1
  Data Type Conversion/1 -> Data Type Duplicate/2, Mux/2

== system hwTarget/hwTarget/GaussianFilter/Symmetric Filter/Verticle Filter/Symmetry ==
  data_in : Inport
  Add : Sum  Inputs=|++  AccumDataTypeStr=cap_2  OutDataTypeStr=cap_2  RndMeth=Nearest
  Data Type Duplicate : DataTypeDuplicate
  Data Type Conversion : DataTypeConversion
  Demux : Demux  Outputs=3
  Mux : Mux  Inputs=2
  data_out : Outport
  wires:
  Add/1 -> Data Type Duplicate/1, Mux/1
  data_in/1 -> Demux/1
  Demux/3 -> Add/2
  Demux/1 -> Add/1
  Mux/1 -> data_out/1
  Demux/2 -> Data Type Conversion/1
  Data Type Conversion/1 -> Data Type Duplicate/2, Mux/2

== system hwTarget/hwTarget/Ix//Iy Filters/Ix Filter/Filter/slicer ==
  note: A|B|C
  note: D|E|F
  note: G|H|I
  data_in : Inport
  Delay{1..6} (6 alike) : Delay  DelayLength=1  InitialCondition=0
  Line buffer : Delay  DelayLength=COLS-2  InitialCondition=0
  Line buffer1 : Delay  DelayLength=COLS-2  InitialCondition=0
  Mux1 : Mux  Inputs=3
  Mux2 : Mux  Inputs=3
  Mux3 : Mux  Inputs=3
  Row1 : Outport  VectorParamsAs1DForOutWhenUnconnected=off
  Row2 : Outport  Port=2  VectorParamsAs1DForOutWhenUnconnected=off
  Row3 : Outport  Port=3  VectorParamsAs1DForOutWhenUnconnected=off
  wires:
  Delay4/1 -> Mux3/3, Line buffer/1
  data_in/1 -> Mux3/1, Delay1/1
  Delay1/1 -> Mux3/2, Delay4/1
  Delay3/1 -> Mux2/2, Delay6/1
  Delay5/1 -> Mux1/3, Line buffer1/1
  Delay6/1 -> Mux2/3
  Line buffer/1 -> Mux1/1, Delay2/1
  Line buffer1/1 -> Mux2/1, Delay3/1
  Delay2/1 -> Mux1/2, Delay5/1
  Mux1/1 -> Row2/1
  Mux2/1 -> Row3/1
  Mux3/1 -> Row1/1

== system hwTarget/hwTarget/Ix//Iy Filters/Iy Filter/Filter/slicer ==
  note: A|B|C
  note: D|E|F
  note: G|H|I
  data_in : Inport
  Delay{1..6} (6 alike) : Delay  DelayLength=1  InitialCondition=0
  Line buffer : Delay  DelayLength=COLS-2  InitialCondition=0
  Line buffer1 : Delay  DelayLength=COLS-2  InitialCondition=0
  Mux1 : Mux  Inputs=3
  Mux2 : Mux  Inputs=3
  Mux3 : Mux  Inputs=3
  Row1 : Outport  VectorParamsAs1DForOutWhenUnconnected=off
  Row2 : Outport  Port=2  VectorParamsAs1DForOutWhenUnconnected=off
  Row3 : Outport  Port=3  VectorParamsAs1DForOutWhenUnconnected=off
  wires:
  Delay4/1 -> Mux3/3, Line buffer/1
  data_in/1 -> Mux3/1, Delay1/1
  Delay1/1 -> Mux3/2, Delay4/1
  Delay3/1 -> Mux2/2, Delay6/1
  Delay5/1 -> Mux1/3, Line buffer1/1
  Delay6/1 -> Mux2/3
  Line buffer/1 -> Mux1/1, Delay2/1
  Line buffer1/1 -> Mux2/1, Delay3/1
  Delay2/1 -> Mux1/2, Delay5/1
  Mux1/1 -> Row2/1
  Mux2/1 -> Row3/1
  Mux3/1 -> Row1/1

== system hwTarget/hwTarget/Kirsch Operation North/Binarize/Subsystem/MagThrL ==
  mean : Inport
  stddev : Inport  Port=2
  dev_step : Inport  Port=3
  Add1 : Sum
  Product : Product
  thresh : Outport
  wires:
  stddev/1 -> Product/1
  mean/1 -> Add1/1
  dev_step/1 -> Product/2
  Product/1 -> Add1/2
  Add1/1 -> thresh/1

== system hwTarget/hwTarget/Kirsch Operation North/Binarize/Subsystem/MagThrS ==
  mean : Inport
  stddev : Inport  Port=2
  dev_step : Inport  Port=3
  Add1 : Sum
  Product : Product
  thresh : Outport
  wires:
  stddev/1 -> Product/1
  mean/1 -> Add1/1
  dev_step/1 -> Product/2
  Product/1 -> Add1/2
  Add1/1 -> thresh/1

== system hwTarget/hwTarget/Kirsch Operation North/Kirch Filter North/Kirch Filter/slicer ==
  note: 5 | 5 | 5
      | -3 | 0 |-3
      | -3 |-3 |-3
  data_in : Inport
  Delay{1..6} (6 alike) : Delay  DelayLength=1  InitialCondition=0
  Display : Display
  Display1 : Display
  Line buffer : Delay  DelayLength=COLS-2  InitialCondition=0
  Line buffer1 : Delay  DelayLength=COLS-2  InitialCondition=0
  Mux : Mux  Inputs=3
  Mux1 : Mux  Inputs=5
  Fives : Outport
  nThrees : Outport  Port=2
  wires:
  Delay4/1 -> Mux1/3, Line buffer/1
  data_in/1 -> Mux1/5, Delay1/1
  Delay1/1 -> Mux1/4, Delay4/1
  Delay3/1 -> Mux/2, Delay6/1
  Delay5/1 -> Line buffer1/1, Mux1/1
  Line buffer/1 -> Mux1/2, Delay2/1
  Line buffer1/1 -> Mux/3, Delay3/1
  Delay2/1 -> Delay5/1
  Mux/1 -> Display1/1, Fives/1
  Mux1/1 -> Display/1, nThrees/1
  Delay6/1 -> Mux/1

== system hwTarget/hwTarget/Kirsch Operation Northwest/Binarize/Subsystem/MagThrL ==
  mean : Inport
  stddev : Inport  Port=2
  dev_step : Inport  Port=3
  Add1 : Sum
  Product : Product
  thresh : Outport
  wires:
  stddev/1 -> Product/1
  mean/1 -> Add1/1
  dev_step/1 -> Product/2
  Product/1 -> Add1/2
  Add1/1 -> thresh/1

== system hwTarget/hwTarget/Kirsch Operation Northwest/Binarize/Subsystem/MagThrS ==
  mean : Inport
  stddev : Inport  Port=2
  dev_step : Inport  Port=3
  Add1 : Sum
  Product : Product
  thresh : Outport
  wires:
  stddev/1 -> Product/1
  mean/1 -> Add1/1
  dev_step/1 -> Product/2
  Product/1 -> Add1/2
  Add1/1 -> thresh/1
